simulink model "runSfunWithCoeffs"  (R2019b)
settings: Solver=FixedStepDiscrete  StartTime=0.0  StopTime=2.0  FixedStep=Ts  RelTol=1e-3  EnableMultiTasking=on
undefined symbols (not defined in the file or in its folder): corrC1, corrC2, corrLength, corrX, corrY, egoTheta, egoX, egoY
settings Model: PauseTimes=341.0  Creator=btc2abt  LastModifiedBy=DOT1BP
settings DataIOCC: LimitDataPoints=on  ReturnWorkspaceOutputs=off
settings OptimizationCC: LifeSpan=inf
settings DebuggingCC: MultiTaskRateTransMsg=warning  AllowSymbolicDim=off  SFUnexpectedBacktrackingDiag=warning  SFNoUnconditionalDefaultTransitionDiag=warning  SFExecutionAtInitializationDiag=none  ArithmeticOperatorsInVariantConditions=warning
settings ModelReferenceCC: PropagateSignalLabelsOutOfModel=off
settings SFSimCC: SimUseLocalCustomCode=off  CustomCodeUndefinedFunction=UseInterfaceOnly
settings RTWCC: RTWUseLocalCustomCode=off
settings CodeAppCC: StateflowObjectComments=on
settings GRTTargetCC: TargetLangStandard=C89/C90 (ANSI)
settings ConfigComp: CovMetricSettings=dw  CovHtmlReporting=on  CovSaveCumulativeToWorkspaceVar=on  CovSaveSingleToWorkspaceVar=on  CovExternalEMLEnable=off

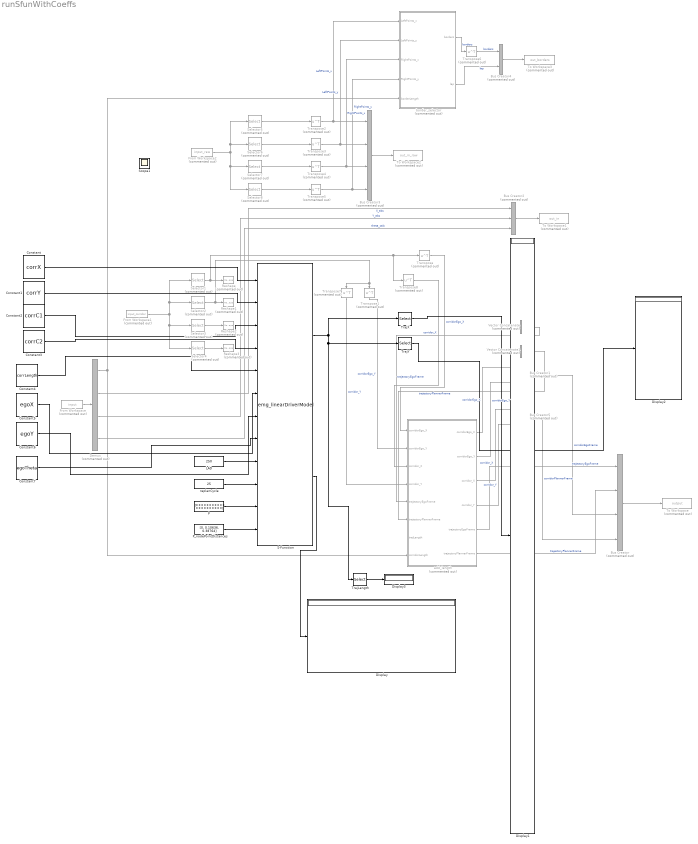
== system runSfunWithCoeffs ==
  Bus Creator : BusCreator  Commented=on  Inputs=4
  Bus Creator1 : BusCreator  Commented=on  Inputs=2
  Bus Creator2 : BusCreator  Commented=on  Inputs=3
  Bus Creator3 : BusCreator  Commented=on  Inputs=4
  Bus Creator4 : BusCreator  Commented=on  Inputs=2
  Bus Creator5 : BusCreator  Commented=on  Inputs=2
  Constant : Constant  Value=corrX
  Constant1 : Constant  Value=corrY
  Constant2 : Constant  Value=corrC1
  Constant3 : Constant  Value=corrC2
  Constant4 : Constant  Value=corrLength
  Constant5 : Constant  Value=egoX
  Constant6 : Constant  Value=egoY
  Constant7 : Constant  Value=egoTheta
  Demux : Demux  Commented=on
  Display{,1..3} (4 alike) : Display
  From Workspace : FromWorkspace  Commented=on  VariableName=input  SampleTime=0  Interpolate=off  OutputAfterFinalValue=Holding final value
  From Workspace1 : FromWorkspace  Commented=on  VariableName=input_corridor  SampleTime=0  Interpolate=off  OutputAfterFinalValue=Holding final value
  From Workspace2 : FromWorkspace  Commented=on  VariableName=input_raw  SampleTime=0
  LAD : Constant  Value=250
  P : Constant  Value=[0 0 0 0 0 0 0 0 0 0 0 0 0 0 0 0 0 0 0 0 0]
  P_nodePointDistances : Constant  Value=[0, 0.10636, 0.38764]
  Reshape{,1..3} (4 alike) : Reshape  Commented=on
  S-Function : S-Function  FunctionName=emg_linearDriverModel  SFunctionDeploymentMode=off  EnableBusSupport=off
  Selector1 : Selector  Commented=on  NumberOfDimensions=2  InputPortWidth=3  IndexOptions=Index vector (dialog),Select all  Indices=[1],1  OutputSizes=1,1
  Selector2 : Selector  Commented=on  NumberOfDimensions=2  InputPortWidth=3  IndexOptions=Index vector (dialog),Select all  Indices=[2],1  OutputSizes=1,1
  Selector3 : Selector  Commented=on  NumberOfDimensions=2  InputPortWidth=3  IndexOptions=Index vector (dialog),Select all  Indices=[3],1  OutputSizes=1,1
  Selector4 : Selector  Commented=on  NumberOfDimensions=2  InputPortWidth=3  IndexOptions=Index vector (dialog),Select all  Indices=[4],1  OutputSizes=1,1
  Selector5 : Selector  Commented=on  NumberOfDimensions=2  InputPortWidth=3  IndexOptions=Index vector (dialog),Select all  Indices=[1],1  OutputSizes=1,1
  Selector6 : Selector  Commented=on  NumberOfDimensions=2  InputPortWidth=3  IndexOptions=Index vector (dialog),Select all  Indices=[2],1  OutputSizes=1,1
  Selector7 : Selector  Commented=on  NumberOfDimensions=2  InputPortWidth=3  IndexOptions=Index vector (dialog),Select all  Indices=[3],1  OutputSizes=1,1
  Selector8 : Selector  Commented=on  NumberOfDimensions=2  InputPortWidth=3  IndexOptions=Index vector (dialog),Select all  Indices=[4],1  OutputSizes=1,1
  To Workspace : ToWorkspace  Commented=on  VariableName=output  SaveFormat=Timeseries  SampleTime=-1
  To Workspace1 : ToWorkspace  Commented=on  VariableName=out_in  SaveFormat=Timeseries  SampleTime=-1
  To Workspace2 : ToWorkspace  Commented=on  VariableName=out_in_raw  SaveFormat=Timeseries  SampleTime=-1
  To Workspace3 : ToWorkspace  Commented=on  VariableName=out_borders  SaveFormat=Timeseries  SampleTime=-1
  TrajLength : Selector  InputPortWidth=601  IndexOptions=Index vector (dialog)  Indices=601  OutputSizes=1
  TrajX : Selector  InputPortWidth=601  IndexOptions=Index vector (dialog)  Indices=linspace(1,300,300)  OutputSizes=1
  TrajY : Selector  InputPortWidth=601  IndexOptions=Index vector (dialog)  Indices=linspace(301,600,300)  OutputSizes=1
  Transpose{,1..8} (9 alike) : Math  Commented=on  Operator=transpose  SignedPower=off  SaturateOnIntegerOverflow=on
  Vector Concatenate : Concatenate  Commented=on  Mode=Multidimensional array  ConcatenateDimension=2
  Vector Concatenate1 : Concatenate  Commented=on  Mode=Multidimensional array  ConcatenateDimension=2
  add_length : MATLAB Function  Commented=on  TreatAsAtomicUnit=on
  border_selector : MATLAB Function  Commented=on  TreatAsAtomicUnit=on
  replanCycle : Constant  Value=25
  Scope1 : Scope
  wires:
  P/1 -> S-Function/11
  P_nodePointDistances/1 -> S-Function/12
  replanCycle/1 -> S-Function/10
  LAD/1 -> S-Function/9
  From Workspace/1 -> Demux/1
  From Workspace1/1 -> Selector1/1, Selector2/1, Selector3/1, Selector4/1
  Selector1/1 -> Transpose/1, Transpose8/1, Reshape/1
  Selector2/1 -> Transpose7/1, Transpose1/1, Reshape1/1
  Selector3/1 -> Reshape2/1
  Selector4/1 -> Reshape3/1
  Demux/1 -> border_selector/5(borderLength), add_length/8(corridorLength)
  Demux/2 -> Bus Creator2/1  "X_abs"
  Demux/3 -> Bus Creator2/2  "Y_abs"
  Demux/4 -> Bus Creator2/3  "theta_calc"
  Bus Creator/1 -> To Workspace/1
  Vector Concatenate/1 -> add_length/5("trajectoryEgoFrame ")  "trajectoryEgoFrame"
  ? -> Vector Concatenate1/1, Vector Concatenate/1
  ? -> Vector Concatenate1/2, Vector Concatenate/2
  Transpose/1 -> add_length/1("corridorEgo_X ")  "corridorEgo_X"
  Transpose1/1 -> add_length/2("corridorEgo_Y ")  "corridorEgo_Y"
  Bus Creator2/1 -> To Workspace1/1
  From Workspace2/1 -> Selector8/1, Selector7/1, Selector6/1, Selector5/1
  Selector5/1 -> Transpose2/1
  Selector6/1 -> Transpose3/1
  Selector7/1 -> Transpose4/1
  Selector8/1 -> Transpose5/1
  Transpose2/1 -> Bus Creator3/1, border_selector/1(LeftPoints_x)  "LeftPoints_x"
  Transpose3/1 -> Bus Creator3/2, border_selector/2(LeftPoints_y)  "LeftPoints_y"
  Transpose4/1 -> Bus Creator3/3, border_selector/3(RightPoints_x)  "RightPoints_x"
  Transpose5/1 -> Bus Creator3/4, border_selector/4(RightPoints_y)  "RightPoints_y"
  Bus Creator3/1 -> To Workspace2/1
  Bus Creator4/1 -> To Workspace3/1
  border_selector/1(borders) -> Transpose6/1  "borders"
  Transpose6/1 -> Bus Creator4/1  "borders"
  border_selector/2(lap) -> Bus Creator4/2  "lap"
  Bus Creator5/1 -> Bus Creator/4  "corridorPlannerFrame"
  Bus Creator1/1 -> Bus Creator/3  "corridorEgoFrame"
  Vector Concatenate1/1 -> add_length/6("trajectoryPlannerFrame ")  "trajectoryPlannerFrame"
  Transpose7/1 -> add_length/4("corridor_Y ")  "corridor_Y"
  Transpose8/1 -> add_length/3("corridor_X ")  "corridor_X"
  add_length/1(corridorEgo_X) -> Bus Creator1/1  "corridorEgo_X"
  add_length/2(corridorEgo_Y) -> Bus Creator1/2  "corridorEgo_Y"
  add_length/3(corridor_X) -> Bus Creator5/1  "corridor_X"
  add_length/4(corridor_Y) -> Bus Creator5/2  "corridor_Y"
  add_length/5(trajectoryEgoFrame) -> Bus Creator/1  "trajectoryEgoFrame"
  add_length/6(trajectoryPlannerFrame) -> Bus Creator/2  "trajectoryPlannerFrame"
  Constant/1 -> S-Function/1
  Constant1/1 -> S-Function/2
  Constant2/1 -> S-Function/3
  Constant3/1 -> S-Function/4
  Constant4/1 -> S-Function/5
  Constant5/1 -> S-Function/6
  Constant6/1 -> S-Function/7
  Constant7/1 -> S-Function/8
  S-Function/2 -> Display/1
  S-Function/1 -> TrajX/1, TrajY/1, TrajLength/1
  TrajLength/1 -> Display3/1
  TrajX/1 -> Display1/1
  TrajY/1 -> Display2/1

== matlab function runSfunWithCoeffs/add_length ==
  data: corridorEgo_X output; corridorEgo_Y output; corridor_X output; corridor_Y output; trajectoryEgoFrame output; trajectoryPlannerFrame output; corridorEgo_X input; corridorEgo_Y input; corridor_X input; corridor_Y input; trajectoryEgoFrame input; trajectoryPlannerFrame input; trajLength input; corridorLength input
function [corridorEgo_X, corridorEgo_Y, corridor_X, corridor_Y, trajectoryEgoFrame, trajectoryPlannerFrame] = add_length(corridorEgo_X, corridorEgo_Y, corridor_X, corridor_Y, trajectoryEgoFrame, trajectoryPlannerFrame, trajLength, corridorLength)

corridorEgo_X(300) = corridorLength;
corridorEgo_Y(300) = corridorLength;
corridor_X(300) = corridorLength;
corridor_Y(300) = corridorLength;
trajectoryEgoFrame(300,:) = trajLength;
trajectoryPlannerFrame(300,:) = trajLength;

end

== matlab function runSfunWithCoeffs/border_selector ==
  data: LeftPoints_x input; borders output; LeftPoints_y input; RightPoints_x input; RightPoints_y input; borderLength input; lap output
function [borders, lap]  = fcn(LeftPoints_x, LeftPoints_y, RightPoints_x, RightPoints_y, borderLength)

lap = zeros(1,3);
borders = zeros(1,82);

borders(1,1:2:39) = LeftPoints_x(1:20);
borders(1,2:2:40) = LeftPoints_y(1:20);
borders(1,42:2:80) = RightPoints_x(1:20);
borders(1,43:2:81) = RightPoints_y(1:20);

borders(1,41) = borderLength;
borders(1,82) = borderLength;

end
